simulink model "RobotinoBahnplanungGesamt_2015b"  (R2015b)
settings: Solver=VariableStepAuto  StartTime=0.0  StopTime=100.0  RelTol=1e-3
undefined symbols (not defined in the file or in its folder): sigbuilder_block
libraries: simulink x3
settings Model: Creator=atlabor  LastModifiedBy=Robin
settings ConfigComp: CovModelRefEnable=Off

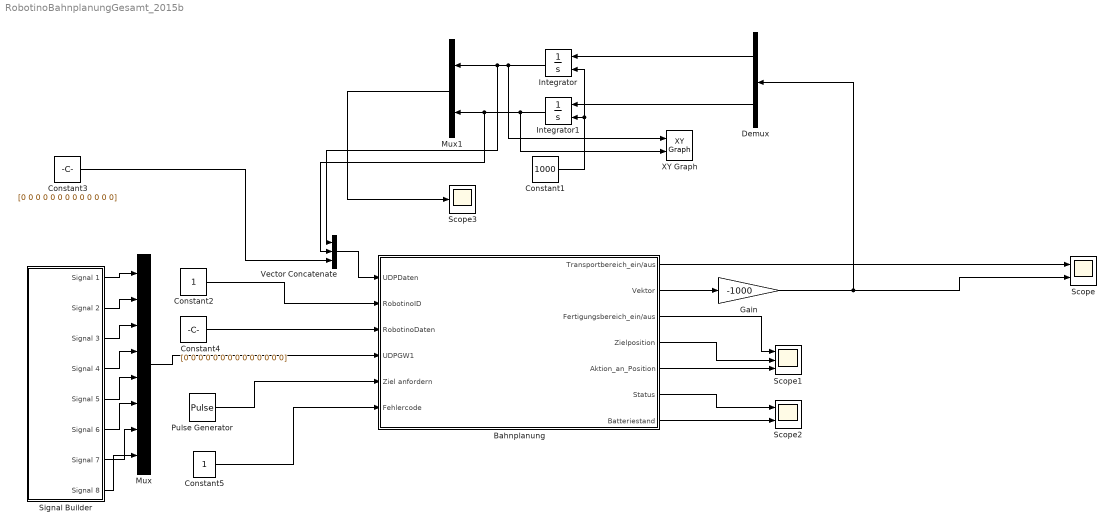
== system RobotinoBahnplanungGesamt_2015b ==
  Bahnplanung : Subsystem
  Constant1 : Constant  Value=1000
  Constant2 : Constant
  Constant3 : Constant  Value=[0 0 0 0 0 0 0 0 0 0 0 0 0]
  Constant4 : Constant  Value=[0 0 0 0 0 0 0 0 0 0 0 0 0 0]
  Constant5 : Constant
  Demux : Demux  Outputs=2
  Gain : Gain  Gain=-1000
  Integrator : Integrator  InitialConditionSource=external
  Integrator1 : Integrator  InitialConditionSource=external
  Mux : Mux  Inputs=8
  Mux1 : Mux  Inputs=2
  Pulse Generator : DiscretePulseGenerator  PulseType=Time based  Period=5  PulseWidth=50
  Scope : Scope  NumInputPorts=2
  Scope1 : Scope  NumInputPorts=3
  Scope2 : Scope  NumInputPorts=2
  Scope3 : Scope
  Signal Builder : Subsystem  Tag=STV Subsys  LoadFcn=sigbuilder_block('load',[0 30 1024.5 488.25 ]);  StartFcn=sigbuilder_block('start');  StopFcn=sigbuilder_block('stop');  ClipboardFcn=sigbuilder_block('clipboard');  mask(Sigbuilder block){}
      mask help: Simulink:masks:SigbuilderBlock_MD
      mask init:
      | if ~strcmp(get_param(bdroot(gcbh),'SimulationStatus'),'stopped') tuvar = sigbuilder_block('maskInit'); end
      settings: CopyFcn=sigbuilder_block('copy');  DeleteFcn=sigbuilder_block('delete');  ModelCloseFcn=sigbuilder_block('modelClose');  PreSaveFcn=sigbuilder_block('preSave');  PauseFcn=sigbuilder_block('pause');  ContinueFcn=sigbuilder_block('continue');  NameChangeFcn=sigbuilder_block('namechange');  OpenFcn=sigbuilder_block('open',[437.6 199.2 550.4 400 ]);  CloseFcn=sigbuilder_block('close');
      mask Display: plot(0, 0, 100, 100,[2, 2, 32, 32, 2], [68, 8, 8, 68, 68],[32, 2], [38, 38], [32, 19, 2],[53, 60, 44], [32, 17, 17, 2],[16, 16, 31, 31]);txt = getActiveGroup(gcbh);text(2, 100, txt,'verticalAlignment', 'top');
  Vector Concatenate : Concatenate  NumInputs=3
  XY Graph : simulink/Sinks/XY Graph  xmin=-1  xmax=5000  ymin=-1  ymax=3000  st=-1
  wires:
  Constant2/1 -> Bahnplanung/2(RobotinoID)
  Mux/1 -> Bahnplanung/4(UDPGW1)
  Bahnplanung/1(Transportbereich_ein/aus) -> Scope/1
  Bahnplanung/3(Fertigungsbereich_ein/aus) -> Scope1/1
  Bahnplanung/4(Zielposition) -> Scope1/2
  Bahnplanung/5(Aktion_an_Position) -> Scope1/3
  Bahnplanung/6(Status) -> Scope2/1
  Bahnplanung/7(Batteriestand) -> Scope2/2
  Constant4/1 -> Bahnplanung/3(RobotinoDaten)
  Constant5/1 -> Bahnplanung/6(Fehlercode)
  Pulse Generator/1 -> Bahnplanung/5(Ziel anfordern)
  Signal Builder/1(Signal 1) -> Mux/1
  Signal Builder/2(Signal 2) -> Mux/2
  Signal Builder/3(Signal 3) -> Mux/3
  Signal Builder/4(Signal 4) -> Mux/4
  Signal Builder/5(Signal 5) -> Mux/5
  Signal Builder/6(Signal 6) -> Mux/6
  Signal Builder/7(Signal 7) -> Mux/7
  Signal Builder/8(Signal 8) -> Mux/8
  Integrator/1 -> XY Graph/1, Vector Concatenate/1, Mux1/1
  Integrator1/1 -> XY Graph/2, Vector Concatenate/2, Mux1/2
  Demux/1 -> Integrator/1
  Demux/2 -> Integrator1/1
  Bahnplanung/2(Vektor) -> Gain/1
  Constant1/1 -> Integrator1/2, Integrator/2
  Mux1/1 -> Scope3/1
  Constant3/1 -> Vector Concatenate/3
  Vector Concatenate/1 -> Bahnplanung/1(UDPDaten)
  Gain/1 -> Demux/1, Scope/2

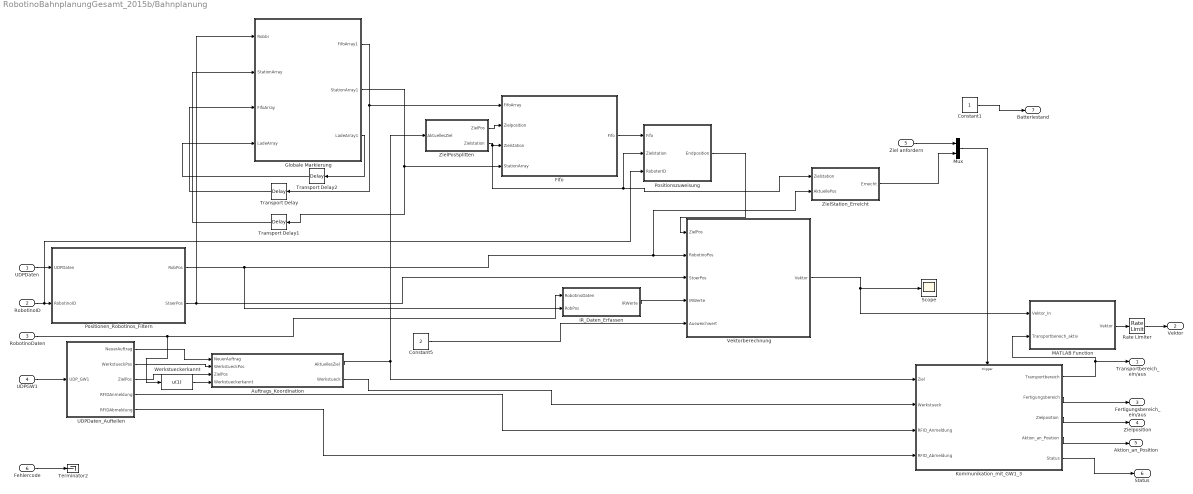
== system RobotinoBahnplanungGesamt_2015b/Bahnplanung ==
  UDPDaten : Inport  PortDimensions=15
  RobotinoID : Inport  Port=2
  RobotinoDaten : Inport  Port=3
  UDPGW1 : Inport  Port=4
  Ziel anfordern : Inport  Port=5
  Fehlercode : Inport  Port=6
  Auftrags_Koordination : Stateflow chart  TreatAsAtomicUnit=on
  Constant1 : Constant
  Constant5 : Constant  Value=2
  Fifo : Stateflow chart  TreatAsAtomicUnit=on
  Globale Markierung : MATLAB Function  TreatAsAtomicUnit=on
  IR_Daten_Erfassen : MATLAB Function  TreatAsAtomicUnit=on
  Kommunikation_mit_GW1_3 : Stateflow chart  TreatAsAtomicUnit=on
  MATLAB Function : MATLAB Function  TreatAsAtomicUnit=on
  Mux : Mux  Inputs=2
  Positionen_Robotinos_Filtern : MATLAB Function  TreatAsAtomicUnit=on
  Positionszuweisung : MATLAB Function  TreatAsAtomicUnit=on
  Rate Limiter : RateLimiter  RisingSlewLimit=0.07  FallingSlewLimit=-0.07  SampleTimeMode=inherited
  Scope : Scope
  Terminator2 : Terminator
  Transport Delay : TransportDelay
  Transport Delay1 : TransportDelay
  Transport Delay2 : TransportDelay
  UDPDaten_Aufteilen : Subsystem
  Vektorberechnung : MATLAB Function  TreatAsAtomicUnit=on
  Werkstueckerkannt : Fcn  Expr=u(1)
  ZielPosSplitten : MATLAB Function  TreatAsAtomicUnit=on
  ZielStation_Erreicht : MATLAB Function  TreatAsAtomicUnit=on
  Transportbereich_ein/aus : Outport
  Vektor : Outport  Port=2  PortDimensions=[1 2]
  Fertigungsbereich_ein/aus : Outport  Port=3
  Zielposition : Outport  Port=4
  Aktion_an_Position : Outport  Port=5
  Status : Outport  Port=6
  Batteriestand : Outport  Port=7
  wires:
  RobotinoID/1 -> Positionszuweisung/3(RoboterID), Positionen_Robotinos_Filtern/2(RobotinoID)
  UDPDaten/1 -> Positionen_Robotinos_Filtern/1(UDPDaten)
  Positionen_Robotinos_Filtern/2(StoerPos) -> Vektorberechnung/3(StoerPos), Globale Markierung/1(Robbi)
  Constant5/1 -> Vektorberechnung/5(Ausweichwert)
  Globale Markierung/2(StationArray1) -> Transport Delay1/1, Fifo/4(StationArray)
  Globale Markierung/1(FifoArray1) -> Transport Delay/1, Fifo/1(FifoArray)
  IR_Daten_Erfassen/1(IRWerte) -> Vektorberechnung/4(IRWerte)
  RobotinoDaten/1 -> IR_Daten_Erfassen/1(RobotinoDaten), Werkstueckerkannt/1
  Kommunikation_mit_GW1_3/3(Zielposition) -> Zielposition/1
  Kommunikation_mit_GW1_3/4(Aktion_an_Position) -> Aktion_an_Position/1
  Kommunikation_mit_GW1_3/2(Fertigungsbereich) -> Fertigungsbereich_ein/aus/1
  Kommunikation_mit_GW1_3/1(Transportbereich) -> Transportbereich_ein/aus/1, MATLAB Function/2(Transportbereich_aktiv)
  Vektorberechnung/1(Vektor) -> Scope/1, MATLAB Function/1(Vektor_In)
  UDPGW1/1 -> UDPDaten_Aufteilen/1(UDP_GW1)
  UDPDaten_Aufteilen/4(RFIDAnmeldung) -> Kommunikation_mit_GW1_3/3(RFID_Anmeldung)
  UDPDaten_Aufteilen/5(RFIDAbmeldung) -> Kommunikation_mit_GW1_3/4(RFID_Abmeldung)
  UDPDaten_Aufteilen/2(WerkstueckPos) -> Auftrags_Koordination/2(WerkstueckPos)
  UDPDaten_Aufteilen/3(ZielPos) -> Auftrags_Koordination/3(ZielPos)
  Auftrags_Koordination/1(AktuellesZiel) -> ZielPosSplitten/1(AktuellesZiel), Kommunikation_mit_GW1_3/1(Ziel)
  ZielPosSplitten/1(ZielPos) -> Fifo/2(Zielposition)
  ZielPosSplitten/2(Zielstation) -> ZielStation_Erreicht/1(Zielstation), Positionszuweisung/2(Zielstation), Fifo/3(Zielstation)
  Fehlercode/1 -> Terminator2/1
  UDPDaten_Aufteilen/1(NeuerAuftrag) -> Auftrags_Koordination/1(NeuerAuftrag)
  Auftrags_Koordination/2(Werkstueck) -> Kommunikation_mit_GW1_3/2(Werkstueck)
  Werkstueckerkannt/1 -> Auftrags_Koordination/4(Werkstueckerkannt)
  Constant1/1 -> Batteriestand/1
  Transport Delay/1 -> Globale Markierung/3(FifoArray)
  Transport Delay1/1 -> Globale Markierung/2(StationArray)
  Fifo/1(Fifo) -> Positionszuweisung/1(Fifo)
  Positionszuweisung/1(Endposition) -> Vektorberechnung/1(ZielPos)
  Kommunikation_mit_GW1_3/5(Status) -> Status/1
  Globale Markierung/3(LadeArray1) -> Transport Delay2/1
  Transport Delay2/1 -> Globale Markierung/4(LadeArray)
  Mux/1 -> Kommunikation_mit_GW1_3/Trigger
  Ziel anfordern/1 -> Mux/1
  ZielStation_Erreicht/1(Erreicht) -> Mux/2
  Positionen_Robotinos_Filtern/1(RobPos) -> IR_Daten_Erfassen/2(RobPos), ZielStation_Erreicht/2(AktuellePos), Vektorberechnung/2(RobotinoPos)
  MATLAB Function/1(Vektor) -> Rate Limiter/1
  Rate Limiter/1 -> Vektor/1

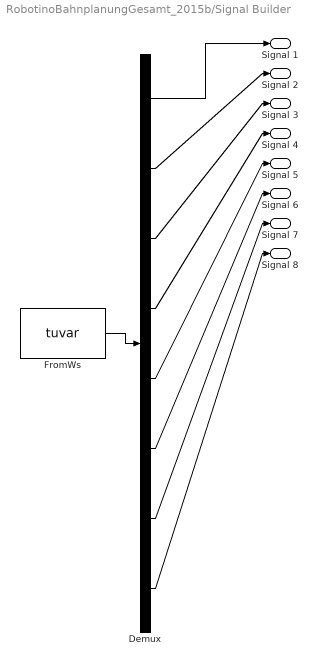
== system RobotinoBahnplanungGesamt_2015b/Signal Builder ==
  Demux : Demux  Tag=STV Demux  Outputs=8
  FromWs : FromWorkspace  Tag=STV FromWs  VariableName=tuvar  SampleTime=0
      SigBuilderData=|
      | common.afterFinalStr = 'Extrapolate'
      | common.sampleTime = 0
      | dataSet.timeRange = [0 10]
      | dataSet.name = 'Group 1'
      | sbobj.Groups.Name = 'Group 1'
      | sbobj.Groups.Signals(1).Name = 'Signal 1'
      | sbobj.Groups.Signals(1).XData = [0 10]
      | sbobj.Groups.Signals(1).YData = [0 0]
      | sbobj.Groups.Signals(2).Name = 'Signal 2'
      | sbobj.Groups.Signals(2).XData = [0 10]
      | sbobj.Groups.Signals(2).YData = [0 0]
      | sbobj.Groups.Signals(3).Name = 'Signal 3'
      | sbobj.Groups.Signals(3).XData = [0 1 1 10]
      | sbobj.Groups.Signals(3).YData = [0 0 1 1]
      | sbobj.Groups.Signals(4).Name = 'Signal 4'
      | sbobj.Groups.Signals(4).XData = [0 1 1 10]
      | sbobj.Groups.Signals(4).YData = [0 0 3 3]
      | sbobj.Groups.Signals(5).Name = 'Signal 5'
      | sbobj.Groups.Signals(5).XData = [0 1 1 10]
      | sbobj.Groups.Signals(5).YData = [0 0 1 1]
      | sbobj.Groups.Signals(6).Name = 'Signal 6'
      | sbobj.Groups.Signals(6).XData = [0 1 1 10]
      | sbobj.Groups.Signals(6).YData = [0 0 1 1]
      | sbobj.Groups.Signals(7).Name = 'Signal 7'
      | sbobj.Groups.Signals(7).XData = [0 1 10]
      | sbobj.Groups.Signals(7).YData = [0 0 0]
      | sbobj.Groups.Signals(8).Name = 'Signal 8'
      | sbobj.Groups.Signals(8).XData = [0 1 1 10]
      | sbobj.Groups.Signals(8).YData = [0 0 3 3]
  Signal 1 : Outport  Tag=STV Outport
  Signal 2 : Outport  Tag=STV Outport  Port=2
  Signal 3 : Outport  Tag=STV Outport  Port=3
  Signal 4 : Outport  Tag=STV Outport  Port=4
  Signal 5 : Outport  Tag=STV Outport  Port=5
  Signal 6 : Outport  Tag=STV Outport  Port=6
  Signal 7 : Outport  Tag=STV Outport  Port=7
  Signal 8 : Outport  Tag=STV Outport  Port=8
  wires:
  Demux/1 -> Signal 1/1
  FromWs/1 -> Demux/1
  Demux/2 -> Signal 2/1
  Demux/3 -> Signal 3/1
  Demux/4 -> Signal 4/1
  Demux/5 -> Signal 5/1
  Demux/6 -> Signal 6/1
  Demux/7 -> Signal 7/1
  Demux/8 -> Signal 8/1

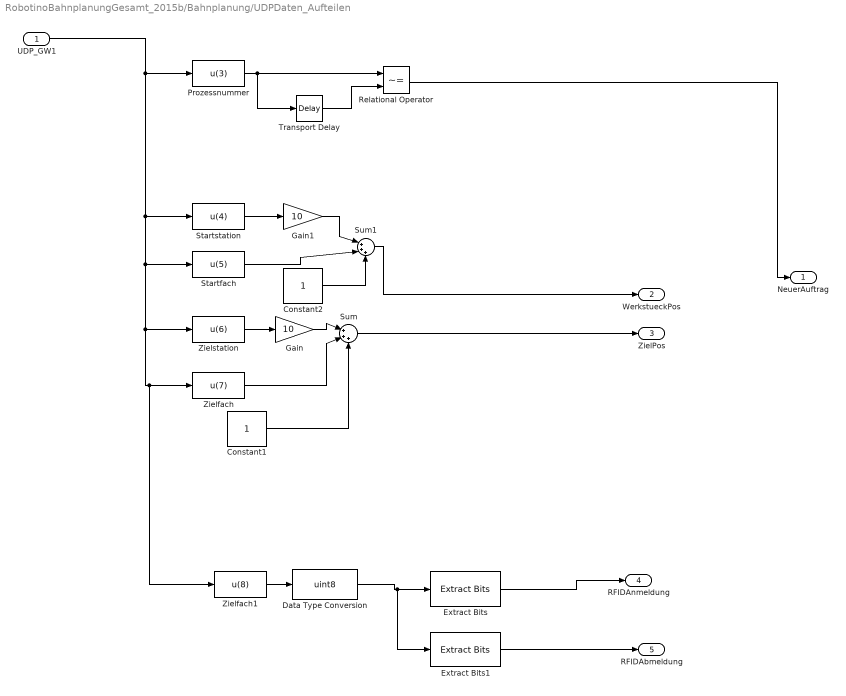
== system RobotinoBahnplanungGesamt_2015b/Bahnplanung/UDPDaten_Aufteilen ==
  UDP_GW1 : Inport
  Constant1 : Constant
  Constant2 : Constant
  Data Type Conversion : DataTypeConversion  OutDataTypeStr=uint8
  Extract Bits : simulink/Logic and Bit Operations/Extract Bits  bitsToExtract=Range of bits  numBits=8  bitIdxRange=[0]  outScalingMode=Treat bit field as an integer
  Extract Bits1 : simulink/Logic and Bit Operations/Extract Bits  bitsToExtract=Range of bits  numBits=8  bitIdxRange=[1]  outScalingMode=Treat bit field as an integer
  Gain : Gain  Gain=10
  Gain1 : Gain  Gain=10
  Prozessnummer : Fcn  Expr=u(3)
  Relational Operator : RelationalOperator  Operator=~=  OutDataTypeStr=boolean
  Startfach : Fcn  Expr=u(5)
  Startstation : Fcn  Expr=u(4)
  Sum : Sum  Inputs=|+++
  Sum1 : Sum  Inputs=|+++
  Transport Delay : TransportDelay
  Zielfach : Fcn  Expr=u(7)
  Zielfach1 : Fcn  Expr=u(8)
  Zielstation : Fcn  Expr=u(6)
  NeuerAuftrag : Outport
  WerkstueckPos : Outport  Port=2
  ZielPos : Outport  Port=3
  RFIDAnmeldung : Outport  Port=4
  RFIDAbmeldung : Outport  Port=5
  wires:
  Zielfach/1 -> Sum/2
  Gain/1 -> Sum/1
  Zielstation/1 -> Gain/1
  UDP_GW1/1 -> Prozessnummer/1, Zielfach1/1, Zielfach/1, Zielstation/1, Startfach/1, Startstation/1
  Sum1/1 -> WerkstueckPos/1
  Startfach/1 -> Sum1/2
  Gain1/1 -> Sum1/1
  Constant2/1 -> Sum1/3
  Startstation/1 -> Gain1/1
  Constant1/1 -> Sum/3
  Sum/1 -> ZielPos/1
  Relational Operator/1 -> NeuerAuftrag/1
  Zielfach1/1 -> Data Type Conversion/1
  Data Type Conversion/1 -> Extract Bits1/1, Extract Bits/1
  Prozessnummer/1 -> Transport Delay/1, Relational Operator/1
  Transport Delay/1 -> Relational Operator/2
  Extract Bits1/1 -> RFIDAbmeldung/1
  Extract Bits/1 -> RFIDAnmeldung/1

== matlab function RobotinoBahnplanungGesamt_2015b/Bahnplanung/Vektorberechnung ==
  data: ZielPos input; Vektor output; RobotinoPos input; StoerPos input; IRWerte input; Ausweichwert input
function Vektor = fcn(ZielPos, RobotinoPos, StoerPos, IRWerte, Ausweichwert)
Stationen=[1103,2308,3507,4694,6300,6300;
            2832,2832,2832,2832,2608,3085;];
Vektor=zeros([1 2]);
K=400;
sigma=187;
SVX=zeros([1 6]);
SVY=zeros([1 6]);
for x=1:6
SVX(x)= -K*exp(-((RobotinoPos(1)-Stationen(1,x))^2+(RobotinoPos(2)-Stationen(2,x))^2)/(2*(sigma^2)))*((RobotinoPos(1)-Stationen(1,x))/(sigma^2));
SVY(x)= -K*exp(-((RobotinoPos(1)-Stationen(1,x))^2+(RobotinoPos(2)-Stationen(2,x))^2)/(2*(sigma^2)))*((RobotinoPos(2)-Stationen(2,x))/(sigma^2));
end
K=0.2;

ZVX = K*(RobotinoPos(1)-ZielPos(1))/sqrt((RobotinoPos(1)-ZielPos(1))^2 +(RobotinoPos(2)-ZielPos(2))^2);
ZVY = K*(RobotinoPos(2)-ZielPos(2))/sqrt((RobotinoPos(1)-ZielPos(1))^2 +(RobotinoPos(2)-ZielPos(2))^2);

K=100;
sigma=224;
RVX=zeros([1 4]);
RVY=zeros([1 4]);
for x=1:4
RVX(x)=-K*exp(-((RobotinoPos(1)-StoerPos((x*3)-2))^2+(RobotinoPos(2)-StoerPos((x*3)-1))^2)/(2*(sigma^2)))*((RobotinoPos(1)-StoerPos((x*3)-2))/(sigma^2));
RVY(x)=-K*exp(-((RobotinoPos(1)-StoerPos((x*3)-2))^2+(RobotinoPos(2)-StoerPos((x*3)-1))^2)/(2*(sigma^2)))*((RobotinoPos(1)-StoerPos((x*3)-1))/(sigma^2));
end
K=50;
sigma=200;
for x=1:9
    IRVX=-K*exp(-((RobotinoPos(1)-IRWerte(1,x))^2+(RobotinoPos(2)-IRWerte(1,x))^2)/(2*(sigma^2)))*((RobotinoPos(1)-IRWerte(1,x))/(sigma^2));
    IRVY=-K*exp(-((RobotinoPos(1)-IRWerte(1,x))^2+(RobotinoPos(2)-IRWerte(2,x))^2)/(2*(sigma^2)))*((RobotinoPos(2)-IRWerte(2,x))/(sigma^2));
end
Distanz=sqrt((RobotinoPos(1)-ZielPos(1))^2+(RobotinoPos(2)-ZielPos(2))^2);
MaxDis=300;
if Distanz > MaxDis
Vektor(1) = sum(SVX)+sum(RVX)+ZVX+sum(IRVX);
Vektor(2) = sum(SVY)+sum(RVY)+ZVY+sum(IRVY);
else
Vektor(1) = (sum(SVX)+sum(RVX)+ZVX+sum(IRVX))*Distanz/MaxDis;
Vektor(2) = (sum(SVY)+sum(RVY)+ZVY+sum(IRVY))*Distanz/MaxDis;  
end

== matlab function RobotinoBahnplanungGesamt_2015b/Bahnplanung/Positionen_Robotinos_Filtern ==
  data: UDPDaten input; RobPos output; RobotinoID input; StoerPos output
function [RobPos,StoerPos]      = fcn(UDPDaten , RobotinoID)
StoerPos=zeros([1 15]);
RobPos=zeros([1 3]);
switch RobotinoID
    case 5
        RobPos(1:3) = UDPDaten(13:15);
        StoerPos(1:12)=UDPDaten(1:12);
    case 4
        RobPos(1:3) = UDPDaten(10:12);
        StoerPos(1:9)=UDPDaten(1:9);
        StoerPos(10:12)=UDPDaten(13:15);
    case 3
        RobPos(1:3) = UDPDaten(7:9);
        StoerPos(1:6)=UDPDaten(1:6);
        StoerPos(7:12)=UDPDaten(10:15);
    case 2
        RobPos(1:3) = UDPDaten(4:6);
        StoerPos(1:3)=UDPDaten(1:3);
        StoerPos(4:12)=UDPDaten(7:15);
    case 1
        RobPos(1:3) = UDPDaten(1:3);
        StoerPos(1:12)=UDPDaten(4:15);
end

== matlab function RobotinoBahnplanungGesamt_2015b/Bahnplanung/ZielStation_Erreicht ==
  data: Zielstation input; Erreicht output; AktuellePos input
function Erreicht = fcn(Zielstation , AktuellePos)
X=AktuellePos(1);
Y=AktuellePos(2);
S=round((X-900)/560);
if Y >2300 && X>600 && X < 5200 && S==Zielstation
    Erreicht=1;
else
    Erreicht=0;
end

== matlab function RobotinoBahnplanungGesamt_2015b/Bahnplanung/IR_Daten_Erfassen ==
  data: RobotinoDaten input; IRWerte output; RobPos input
function IRWerte = fcn(RobotinoDaten,RobPos)
IRWerte=zeros([2 9]);
IRDaten=zeros([1 9]);
IRDaten=RobotinoDaten(6:14);

for x=1:9
    IRWerte(1,x)=cos((((x-1)*40)-RobPos(3))*pi/180)*IRDaten(x)+RobPos(1);
    IRWerte(2,x)=sin((((x-1)*40)-RobPos(3))*pi/180)*IRDaten(x)+RobPos(2);
end

== stateflow chart RobotinoBahnplanungGesamt_2015b/Bahnplanung/Kommunikation_mit_GW1_3 ==
  state KommunikationGW3
    state Fertigungsbereich
      entry:Transportbereich=0,
      Fertigungsbereich=1;
      state RFID_einchecken
        entry:Zielposition=Ziel-mod(Ziel,10)+3,
        Aktion_an_Position=Aktion_Warten,
        Status=2;
      state Startpunkt
        entry: Zielposition=Ziel-mod(Ziel,10);
        Aktion_an_Position=Aktion_Warten,
        Status=1;
      state Warten
        entry: BereichVerlassen=1,
        if  Werkstueck==0
        Status=0;
        end
      state Position_anfahren
        entry:Zielposition=Ziel,
        Status=1,
        if Werkstueck==0
        Aktion_an_Position=Aktion_Aufnehmen;
        else
        Aktion_an_Position=Aktion_Ablegen;
        end
      state Bereich_verlassen
        entry:Zielposition=Ziel-mod(Ziel,10)+4,
        Aktion_an_Position=Aktion_Warten,
        Status=1;
      state RFID_auschecken
        entry:Zielposition=Ziel-mod(Ziel,10)+3,
        Aktion_an_Position=Aktion_Warten,
        Status=3;
      Startpunkt -> RFID_einchecken [order 1] : [Ziel_anfordern & Werkstueck==1]
      (default) -> Startpunkt
      RFID_einchecken -> Position_anfahren : [RFID_Anmeldung==1]
      Startpunkt -> Position_anfahren [order 2] : [Ziel_anfordern & Werkstueck==0]
      Bereich_verlassen -> Warten : Ziel_anfordern
      Position_anfahren -> Bereich_verlassen [order 2] : [Ziel_anfordern & (Aktion_an_Position==Aktion_Ablegen)]
      Position_anfahren -> RFID_auschecken [order 1] : [Ziel_anfordern & (Aktion_an_Position==Aktion_Aufnehmen)]
      RFID_auschecken -> Bereich_verlassen : [RFID_Abmeldung==1]
    state Transportbereich
      entry:Transportbereich=1,
      Fertigungsbereich=0,
      BereichVerlassen=0;
    state Init
      entry: Transportbereich=0,
      Fertigungsbereich=0,
      Status=0;
    (default) -> Init
    Transportbereich -> Fertigungsbereich : ZielStation_Erreicht
    Init -> Transportbereich
    Fertigungsbereich -> Transportbereich : [BereichVerlassen==1]
  data: Transportbereich output; Fertigungsbereich output; Ziel input; Zielposition output; Aktion_an_Position output; Aktion_Warten local double =2; Aktion_Aufnehmen local double =1; Aktion_Ablegen local double =0; Werkstueck input double; Wartezeit local double =5; RFID_Anmeldung input; RFID_Abmeldung input; BereichVerlassen local; Status output
  events: Ziel_anfordern input RISING_EDGE_EVENT; ZielStation_Erreicht input RISING_EDGE_EVENT

== stateflow chart RobotinoBahnplanungGesamt_2015b/Bahnplanung/Auftrags_Koordination ==
  settings: updateMethod=DISCRETE  sampleTime=0.01
  state Auftragskoordination
    state WerkstueckAufgenommen
      entry:Werkstueck=1,
      AktuellesZiel=ZielPos;
    state KeinWerkstueckAufgenommen
      entry:Werkstueck=0,
      AktuellesZiel=WerkstueckPos;
    state AufAuftragWarten
      entry:Werkstueck=0,
      AktuellesZiel=100;
    KeinWerkstueckAufgenommen -> WerkstueckAufgenommen : [Werkstueckerkannt==1]
    WerkstueckAufgenommen -> AufAuftragWarten : [Werkstueckerkannt==0]
    AufAuftragWarten -> KeinWerkstueckAufgenommen : [NeuerAuftrag]
    (default) -> AufAuftragWarten
  data: NeuerAuftrag input; WerkstueckPos input; ZielPos input; AktuellesZiel output; Werkstueck output; Werkstueckerkannt input

== matlab function RobotinoBahnplanungGesamt_2015b/Bahnplanung/ZielPosSplitten ==
  data: AktuellesZiel input; ZielPos output; Zielstation output
function [ZielPos,Zielstation]= fcn(AktuellesZiel)
ZielPos=mod(AktuellesZiel,10);
Zielstation=round(AktuellesZiel/10);

== matlab function RobotinoBahnplanungGesamt_2015b/Bahnplanung/MATLAB Function ==
  data: Vektor_In input; Vektor output; Transportbereich_aktiv input
function Vektor = fcn(Vektor_In,Transportbereich_aktiv)
Vektor=zeros([1 2]);
if Transportbereich_aktiv==1
    Vektor=Vektor_In;
end

== stateflow chart RobotinoBahnplanungGesamt_2015b/Bahnplanung/Fifo ==
  settings: updateMethod=DISCRETE  sampleTime=0.01
  state FIFOStationen
    state Auftrag_Roboter_1
    state Zielbereich_untersuchen
      entry:
      ersterFifo=floor(Zielstation/2)*3+2*mod(Zielstation,2);
    state Fifo_einfachbesetzt1
      entry:
      zweiterFifo=floor(Zielstation/2)*3+1;
      Fifo=2;
    state Fifo_frei
      entry:
      Fifo=1;
    state Fifo_doppelt_besetzt
      entry:
      dritterFifo=floor(Zielstation/2)*3+2-2*mod(Zielstation,2);
      Fifo=3;
    state Fifo_voll
      entry:
      Fifo=4;
    state Uebergabepunkt_gleich_Zielpunkt
      entry:
      Fifo=0;
    (default) -> Auftrag_Roboter_1
    Auftrag_Roboter_1 -> Zielbereich_untersuchen : [Zielposition>-1]
    Zielbereich_untersuchen -> Fifo_einfachbesetzt1 [order 1] : [(FifoArray(ersterFifo)~=0)| (FifoArray(ersterFifo)==0 & StationArray(Zielstation)~=0) ]
    Zielbereich_untersuchen -> Uebergabepunkt_gleich_Zielpunkt [order 2]
    Fifo_einfachbesetzt1 -> Fifo_frei [order 2] : [FifoArray(ersterFifo)==0]
    Fifo_einfachbesetzt1 -> Fifo_doppelt_besetzt [order 1] : [(FifoArray(zweiterFifo)~=0)]
    Fifo_doppelt_besetzt -> Fifo_voll [order 2] : [(FifoArray(dritterFifo)~=0)]
    Fifo_frei -> Uebergabepunkt_gleich_Zielpunkt : [ StationArray(Zielstation)==0]
    Fifo_doppelt_besetzt -> Fifo_einfachbesetzt1 [order 1] : [FifoArray(zweiterFifo)==0]
    Fifo_voll -> Fifo_doppelt_besetzt : [FifoArray(dritterFifo)==0]
  state Wartebereich
    entry: Fifo=4;
  state Ladestation
    entry: Fifo=0;
  (default) -> Wartebereich
  Wartebereich -> FIFOStationen [order 1] : [Zielstation<8]
  FIFOStationen -> Wartebereich [order 1] : [Zielstation==10]
  Ladestation -> Wartebereich [order 1] : [Zielstation==10]
  Wartebereich -> Ladestation [order 2] : [Zielstation>=8 & Zielstation<10]
  Ladestation -> FIFOStationen [order 2] : [Zielstation<8]
  FIFOStationen -> Ladestation [order 2] : [Zielstation>=8 & Zielstation<10]
  data: FifoArray input; Zielposition input; Zielstation input; Fifo output; StationArray input; dritterFifo local; zweiterFifo local; ersterFifo local

== matlab function RobotinoBahnplanungGesamt_2015b/Bahnplanung/Positionszuweisung ==
  data: Fifo input; Zielstation input; Endposition output; RoboterID input
function Endposition = fcn(Fifo,Zielstation,RoboterID)
Endposition=zeros([1 2]);

WartepositionX= 6311;
WartepositionY=[550 950 1350 1750 2150];

StationvorneX=[853 1361 2058 2559 3256 3762 4448 4953 6311 6311];
StationvorneY=[2300 2300 2300 2300 2300 2300 2300 2300 2592 3080];
%Stationhinten=[856 1364 2059 2560 3259 3763 4451 4958];

ersterFifo=floor(Zielstation/2)*3+2*mod(Zielstation,2);
zweiterFifo=floor(Zielstation/2)*3+1;
dritterFifo=floor(Zielstation/2)*3+2-2*mod(Zielstation,2);

if Fifo==0
    Endposition(1)=StationvorneX(Zielstation+1);
    Endposition(2)=StationvorneY(Zielstation+1);
    else if Fifo==1
        Endposition(1)= ersterFifo*400+703;
        Endposition(2)= 250;
       
    else if Fifo==2
            Endposition(1)= zweiterFifo*400+703;
            Endposition(2)= 250;
        
    else if Fifo==3
            Endposition(1)= dritterFifo*400+703;
            Endposition(2)= 250;
            else
            Endposition(2)= WartepositionY(RoboterID);
            Endposition(1)= WartepositionX;
        end
        end
        end
end
end

== matlab function RobotinoBahnplanungGesamt_2015b/Bahnplanung/Globale Markierung ==
  data: Robbi input; StationArray input; FifoArray input; FifoArray1 output; StationArray1 output; LadeArray input; LadeArray1 output
function [FifoArray1,StationArray1,LadeArray1]= fcn(Robbi,StationArray,FifoArray,LadeArray)
X=zeros([1 4]);
Y=zeros([1 4]);
X=[Robbi(1) Robbi(4) Robbi(7) Robbi(10)];
Y=[Robbi(2) Robbi(5) Robbi(8) Robbi(11)];
FifoArray1=zeros([1 12]);
FifoArray1=FifoArray(1:12);
StationArray1=zeros([1 8]);
StationArray1=StationArray(1:8);
LadeArray1=zeros([1 2]);
LadeArray1=LadeArray(1:2);
N=zeros([1 4]);
S=zeros([1 4]);
L=zeros([1 4]);
for n= 1 : 1 : 4
    L(n)=round((Y(n)-2592)/500);
    N(n)=round((X(n)-703)/400);   % Berechnung in welchem Fifo der Roboter sich befindet
    S(n)=round((X(n)-900)/560);   %Berechnung in welcher Station der Roboter sich befindet
     if (X(n)<=6000 || X(n)>6500)
        for i=1:2
            if LadeArray1(i)==n
                LadeArray1(i)=0;
            end
        end
     end
    if (X(n)>6000 && X(n)<=6500 && Y(n)>2300 &&Y(n)<=3300)
        LadeArray1(L(n))=n;
    end  
    if (Y(n)<=2100 || Y(n)>3400)
        for i=1:8
            if StationArray1(i)==n
                StationArray(i)=0;
            end
        end
    end
    if (Y(n)>2100 && X(n)<5100) 
         for i=1:12
            if FifoArray1(i)==n
                FifoArray1(i)=0;
            end
        end
        StationArray1(S(n))=n;
        
    else if (Y(n)<450 && (X(n)>100 && X(n)<5250))
        for i=1:12
            if FifoArray1(i)==n
                FifoArray1(i)=0;
            end
        end
            FifoArray1(N(n))=n;
        end
    end
end
